simulink model "RegenModel"  (R2024b)
settings: Solver=VariableStepAuto  StartTime=0.0  StopTime=10.0  RelTol=1e-1
settings Model: Creator=khalid  LastModifiedBy=khalidwaleed

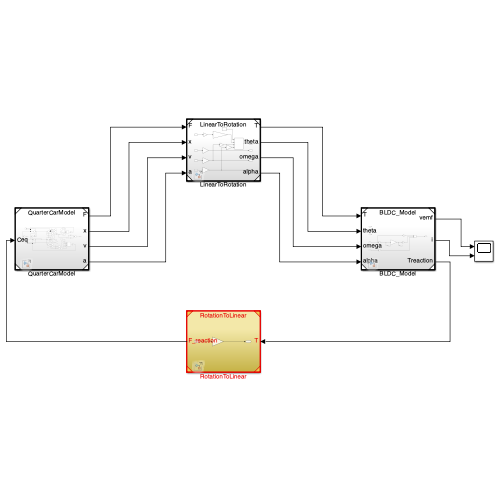
[thumbnail: Simulink's stored preview of the top-level diagram]
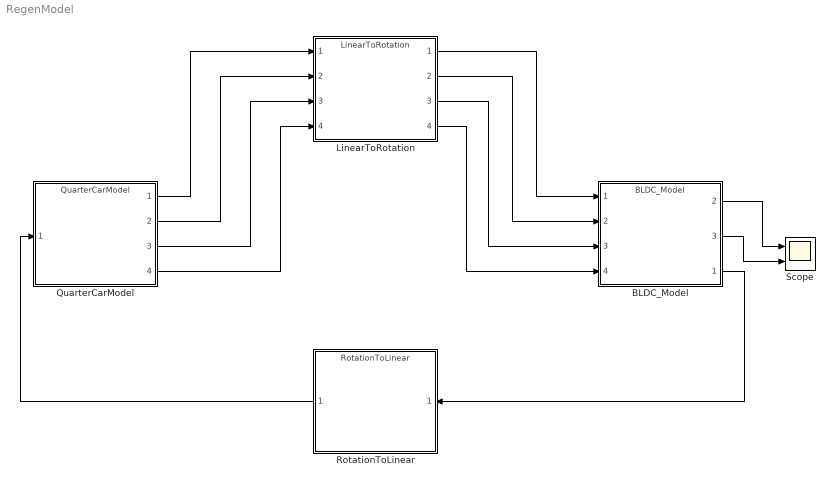
== system RegenModel ==
  BLDC_Model : ModelReference  ModelNameDialog=BLDC_Model.slx  SimulationMode=Normal  ModelReferenceVersion=1.2
      settings: PortSchema="{\"entries\":[{\"content\":{\"sides\":[{\"content\":{\"connectorIds\":[\"In1\",\"In2\",\"In3\",\"In4\"]},\"type\":\"ConnectorPlacement.EquallySpacedRectSide\",\"uuid\":\"70fa63f0-b672-4e1a-963d-5b71f8ee4ba9\"},{\"content\":{\"connectorIds\":[\"Out2\",\"Out3\",\"Out1\"],\"side\":\"RIGHT\"},\"type\":\"ConnectorPlacement.EquallySpacedRectSide\",\"uuid\":\"c947323e-70da-4da4-9287-6c1e8ab1bcfa\"},{\"content\":{\"side\":\"TOP\"},\"type\":\"ConnectorPlacement.EquallySpacedRectSide\",\"uuid\":\"d5e85f82-72aa-46a0-934b-eddab25ffda0\"}]},\"type\":\"ConnectorPlacement.EquallySpacedConnector\",\"uuid\":\"46fba77d-0ac4-43ef-9099-b17e30fa2275\"}],\"packageUris\":[\"http://schema.mathworks.com/mf0/Connector/R2020b\"],\"version\":\"1.0\"}"
  LinearToRotation : ModelReference  ModelNameDialog=LinearToRotation.slx  SimulationMode=Normal  ModelReferenceVersion=1.4
  QuarterCarModel : ModelReference  ModelNameDialog=QuarterCarModel.slx  SimulationMode=Normal  ModelReferenceVersion=1.4
  RotationToLinear : ModelReference  ModelNameDialog=RotationToLinear.slx  SimulationMode=Normal  ModelReferenceVersion=1.2
      settings: PortSchema="{\"entries\":[{\"content\":{\"sides\":[{\"content\":{\"connectorIds\":[\"Out1\"]},\"type\":\"ConnectorPlacement.EquallySpacedRectSide\",\"uuid\":\"0a7b994f-b6f6-4f40-864d-5366077339c7\"},{\"content\":{\"connectorIds\":[\"In1\"],\"side\":\"RIGHT\"},\"type\":\"ConnectorPlacement.EquallySpacedRectSide\",\"uuid\":\"5092f5a5-35c7-40a7-8c19-dd0ec99b0e60\"},{\"content\":{\"side\":\"TOP\"},\"type\":\"ConnectorPlacement.EquallySpacedRectSide\",\"uuid\":\"eb32addd-3f6d-4eda-ab61-3328a41c6b22\"}]},\"type\":\"ConnectorPlacement.EquallySpacedConnector\",\"uuid\":\"9e7435b1-5d6e-4647-ad29-59f13bdef716\"}],\"packageUris\":[\"http://schema.mathworks.com/mf0/Connector/R2020b\"],\"version\":\"1.0\"}"
  Scope : Scope  NumInputPorts=2
  wires:
  QuarterCarModel/1 -> LinearToRotation/1
  QuarterCarModel/2 -> LinearToRotation/2
  QuarterCarModel/3 -> LinearToRotation/3
  QuarterCarModel/4 -> LinearToRotation/4
  LinearToRotation/1 -> BLDC_Model/1
  LinearToRotation/2 -> BLDC_Model/2
  LinearToRotation/4 -> BLDC_Model/4
  BLDC_Model/2 -> Scope/1
  BLDC_Model/3 -> Scope/2
  BLDC_Model/1 -> RotationToLinear/1
  RotationToLinear/1 -> QuarterCarModel/1
  LinearToRotation/3 -> BLDC_Model/3
